simulink model "r2_deng_tvg_rev1_13"  (R2012b)
(part 3 of 65)

      |     mask_enables{ismember(mask_names, 'sample_period')} = 'on';
      | end
      | set_param(gcb, 'MaskEnables', mask_enables);
  speadtime1_offset : Subsystem  Tag=xps:sw_reg  AncestorBlock=xps_library/software register  mask(swreg){io_dir=From Processor, io_delay=1, sample_period=1, names=speadtime_offset1, bitwidths=32, bin_pts=0, arith_types=0, sim_port=on, show_format=on}
      mask prompts: io_dir "I/O direction"; io_delay "I/O delay"; sample_period "Sample period"; names "Bitfield names [msb...lsb]"; bitwidths "Bitfield widths"; bin_pts "Bitfield binary pts"; arith_types "Bitfield types, ufix=0, fix=1, bool=2"; sim_port "Provide sim input/output?"; show_format "Print format string?"
      mask help: A 32-bit software-accessible register. Can be divided into bitfields of varying widths and types using the fields in the block mask.
      mask init:
      | try
      |     swreg_init(gcb)
      | catch ex
      |     disp(sprintf('%s: %s', gcb, ex.message))
      |     errordlg(ex.message)
      | end
      settings: AttributesFormatString=1input:uf32.0 = 32 bits
      mask TypeOptions io_dir: To Processor | From Processor
      mask Callback io_dir:
      | mask_enables = get_param(gcb, 'MaskEnables');
      | mask_names = get_param(gcb, 'MaskNames');
      | if strcmp(get_param(gcb, 'io_dir'), 'To Processor'),
      |     mask_enables{ismember(mask_names, 'sample_period')} = 'off';
      | else
      |     mask_enables{ismember(mask_names, 'sample_period')} = 'on';
      | end
      | set_param(gcb, 'MaskEnables', mask_enables);
  src_sel_cntrl : Subsystem  Tag=xps:sw_reg  AncestorBlock=xps_library/software register  mask(swreg){io_dir=From Processor, io_delay=1, sample_period=1, names=[src_sel_0 src_sel_1], bitwidths=[2 2], bin_pts=[0 0], arith_types=[0 0], sim_port=on, show_format=on}
      mask prompts: io_dir "I/O direction"; io_delay "I/O delay"; sample_period "Sample period"; names "Bitfield names [msb...lsb]"; bitwidths "Bitfield widths"; bin_pts "Bitfield binary pts"; arith_types "Bitfield types, ufix=0, fix=1, bool=2"; sim_port "Provide sim input/output?"; show_format "Print format string?"
      mask help: A 32-bit software-accessible register. Can be divided into bitfields of varying widths and types using the fields in the block mask.
      mask init:
      | try
      |     swreg_init(gcb)
      | catch ex
      |     disp(sprintf('%s: %s', gcb, ex.message))
      |     errordlg(ex.message)
      | end
      settings: AttributesFormatString=2 inputs:uf2.0,uf2.0 = 4 bits
      mask TypeOptions io_dir: To Processor | From Processor
      mask Callback io_dir:
      | mask_enables = get_param(gcb, 'MaskEnables');
      | mask_names = get_param(gcb, 'MaskNames');
      | if strcmp(get_param(gcb, 'io_dir'), 'To Processor'),
      |     mask_enables{ismember(mask_names, 'sample_period')} = 'off';
      | else
      |     mask_enables{ismember(mask_names, 'sample_period')} = 'on';
      | end
      | set_param(gcb, 'MaskEnables', mask_enables);
  ss_fifo_in : Subsystem  Tag=casper:bitsnap  AncestorBlock=casper_library_scopes/bitfield snapshot  mask(bitsnap){io_names=[d0 d1 d2 d3 d4 d5 d6 d7 gpio_trig], io_widths=[10 10 10 10 10 10 10 10 1], io_bps=[9 9 9 9 9 9 9 9 0], io_types=[1 1 1 1 1 1 1 1 2], show_format=on, snap_storage=bram, snap_dram_dimm=2, snap_dram_clock=250, snap_nsamples=9, snap_data_width=128, snap_offset=on, snap_circap=off, snap_value=off, snap_use_dsp48=off, snap_delay=1, extra_names=[c d], extra_widths=[30 2], extra_bps=[0 0], extra_types=[0 0]}
      mask prompts: io_names "Names [msb...lsb]"; io_widths "Bitwidths [msb...lsb]"; io_bps "Binary pts [msb...lsb]"; io_types "Data types [msb...lsb], ufix=0, fix=1, bool=2"; show_format "Print format string?"; snap_storage "Storage medium"; snap_dram_dimm "DRAM dimm"; snap_dram_clock "DRAM clock rate"; snap_nsamples "Number of Samples (2^?)"; snap_data_width "Data width"; snap_offset "Start delay support"; snap_circap "Circular capture support"; snap_value "Extra value capture support"; snap_use_dsp48 "Use DSP48s to implement counters"; snap_delay "Pre-snapshot delay"; extra_names "Names [msb...lsb]"; extra_widths "Widths [msb...lsb]"; extra_bps "Binary pts [msb...lsb]"; extra_types "Data types [msb...lsb], ufix=0, fix=1, bool=2"
      mask help:
      | A wrapped snapshot block. Allows specification of inputs to a snapblock word so the toolflow can automatically set up the scope.
      | See documentation for snapshot for explanation of parameters.
      mask init:
      | bitsnap_init(gcb);
      settings: AttributesFormatString=snap(9):f10.9,f10.9,f10.9,f10.9,f10.9,f10.9,f10.9,f10.9,b = 81 bits
      mask TypeOptions snap_storage: bram | dram
      mask Callback snap_storage: bitsnap_callback();
      mask TypeOptions snap_dram_dimm: 1 | 2 | 3 | 4
      mask TypeOptions snap_dram_clock: 200 | 250 | 266 | 300 | 333
      mask TypeOptions snap_data_width: 8 | 16 | 32 | 64 | 128
      mask Callback snap_value: bitsnap_callback();
  ss_localtime : Subsystem  Tag=casper:bitsnap  AncestorBlock=casper_library_scopes/bitfield snapshot  mask(bitsnap){io_names=time, io_widths=64, io_bps=0, io_types=0, show_format=on, snap_storage=bram, snap_dram_dimm=2, snap_dram_clock=250, snap_nsamples=9, snap_data_width=64, snap_offset=on, snap_circap=off, snap_value=off, snap_use_dsp48=off, snap_delay=1, extra_names=[c d], extra_widths=[30 2], extra_bps=[0 0], extra_types=[0 0]}
      mask prompts: io_names "Names [msb...lsb]"; io_widths "Bitwidths [msb...lsb]"; io_bps "Binary pts [msb...lsb]"; io_types "Data types [msb...lsb], ufix=0, fix=1, bool=2"; show_format "Print format string?"; snap_storage "Storage medium"; snap_dram_dimm "DRAM dimm"; snap_dram_clock "DRAM clock rate"; snap_nsamples "Number of Samples (2^?)"; snap_data_width "Data width"; snap_offset "Start delay support"; snap_circap "Circular capture support"; snap_value "Extra value capture support"; snap_use_dsp48 "Use DSP48s to implement counters"; snap_delay "Pre-snapshot delay"; extra_names "Names [msb...lsb]"; extra_widths "Widths [msb...lsb]"; extra_bps "Binary pts [msb...lsb]"; extra_types "Data types [msb...lsb], ufix=0, fix=1, bool=2"
      mask help:
      | A wrapped snapshot block. Allows specification of inputs to a snapblock word so the toolflow can automatically set up the scope.
      | See documentation for snapshot for explanation of parameters.
      mask init:
      | bitsnap_init(gcb);
      settings: AttributesFormatString=snap(1):uf64.0 = 64 bits
      mask TypeOptions snap_storage: bram | dram
      mask Callback snap_storage: bitsnap_callback();
      mask TypeOptions snap_dram_dimm: 1 | 2 | 3 | 4
      mask TypeOptions snap_dram_clock: 200 | 250 | 266 | 300 | 333
      mask TypeOptions snap_data_width: 8 | 16 | 32 | 64 | 128
      mask Callback snap_value: bitsnap_callback();
  ss_trig_time_lsw : Subsystem  Tag=xps:sw_reg  AncestorBlock=xps_library/software register  mask(swreg){io_dir=From Processor, io_delay=1, sample_period=1, names=reg, bitwidths=32, bin_pts=0, arith_types=0, sim_port=on, show_format=on}
      mask prompts: io_dir "I/O direction"; io_delay "I/O delay"; sample_period "Sample period"; names "Bitfield names [msb...lsb]"; bitwidths "Bitfield widths"; bin_pts "Bitfield binary pts"; arith_types "Bitfield types, ufix=0, fix=1, bool=2"; sim_port "Provide sim input/output?"; show_format "Print format string?"
      mask help: A 32-bit software-accessible register. Can be divided into bitfields of varying widths and types using the fields in the block mask.
      mask init:
      | try
      |     swreg_init(gcb)
      | catch ex
      |     disp(sprintf('%s: %s', gcb, ex.message))
      |     errordlg(ex.message)
      | end
      settings: AttributesFormatString=1input:uf32.0 = 32 bits
      mask TypeOptions io_dir: To Processor | From Processor
      mask Callback io_dir:
      | mask_enables = get_param(gcb, 'MaskEnables');
      | mask_names = get_param(gcb, 'MaskNames');
      | if strcmp(get_param(gcb, 'io_dir'), 'To Processor'),
      |     mask_enables{ismember(mask_names, 'sample_period')} = 'off';
      | else
      |     mask_enables{ismember(mask_names, 'sample_period')} = 'on';
      | end
      | set_param(gcb, 'MaskEnables', mask_enables);
  ss_trig_time_msw : Subsystem  Tag=xps:sw_reg  AncestorBlock=xps_library/software register  mask(swreg){io_dir=From Processor, io_delay=1, sample_period=1, names=reg, bitwidths=32, bin_pts=0, arith_types=0, sim_port=on, show_format=on}
      mask prompts: io_dir "I/O direction"; io_delay "I/O delay"; sample_period "Sample period"; names "Bitfield names [msb...lsb]"; bitwidths "Bitfield widths"; bin_pts "Bitfield binary pts"; arith_types "Bitfield types, ufix=0, fix=1, bool=2"; sim_port "Provide sim input/output?"; show_format "Print format string?"
      mask help: A 32-bit software-accessible register. Can be divided into bitfields of varying widths and types using the fields in the block mask.
      mask init:
      | try
      |     swreg_init(gcb)
      | catch ex
      |     disp(sprintf('%s: %s', gcb, ex.message))
      |     errordlg(ex.message)
      | end
      settings: AttributesFormatString=1input:uf32.0 = 32 bits
      mask TypeOptions io_dir: To Processor | From Processor
      mask Callback io_dir:
      | mask_enables = get_param(gcb, 'MaskEnables');
      | mask_names = get_param(gcb, 'MaskNames');
      | if strcmp(get_param(gcb, 'io_dir'), 'To Processor'),
      |     mask_enables{ismember(mask_names, 'sample_period')} = 'off';
      | else
      |     mask_enables{ismember(mask_names, 'sample_period')} = 'on';
      | end
      | set_param(gcb, 'MaskEnables', mask_enables);
  start_flag_lsw : Subsystem  Tag=xps:sw_reg  AncestorBlock=xps_library/software register  mask(swreg){io_dir=From Processor, io_delay=1, sample_period=1, names=reg, bitwidths=32, bin_pts=0, arith_types=0, sim_port=on, show_format=on}
      mask prompts: io_dir "I/O direction"; io_delay "I/O delay"; sample_period "Sample period"; names "Bitfield names [msb...lsb]"; bitwidths "Bitfield widths"; bin_pts "Bitfield binary pts"; arith_types "Bitfield types, ufix=0, fix=1, bool=2"; sim_port "Provide sim input/output?"; show_format "Print format string?"
      mask help: A 32-bit software-accessible register. Can be divided into bitfields of varying widths and types using the fields in the block mask.
      mask init:
      | try
      |     swreg_init(gcb)
      | catch ex
      |     disp(sprintf('%s: %s', gcb, ex.message))
      |     errordlg(ex.message)
      | end
      settings: AttributesFormatString=1input:uf32.0 = 32 bits
      mask TypeOptions io_dir: To Processor | From Processor
      mask Callback io_dir:
      | mask_enables = get_param(gcb, 'MaskEnables');
      | mask_names = get_param(gcb, 'MaskNames');
      | if strcmp(get_param(gcb, 'io_dir'), 'To Processor'),
      |     mask_enables{ismember(mask_names, 'sample_period')} = 'off';
      | else
      |     mask_enables{ismember(mask_names, 'sample_period')} = 'on';
      | end
      | set_param(gcb, 'MaskEnables', mask_enables);
  start_flag_msw : Subsystem  Tag=xps:sw_reg  AncestorBlock=xps_library/software register  mask(swreg){io_dir=From Processor, io_delay=1, sample_period=1, names=reg, bitwidths=32, bin_pts=0, arith_types=0, sim_port=on, show_format=on}
      mask prompts: io_dir "I/O direction"; io_delay "I/O delay"; sample_period "Sample period"; names "Bitfield names [msb...lsb]"; bitwidths "Bitfield widths"; bin_pts "Bitfield binary pts"; arith_types "Bitfield types, ufix=0, fix=1, bool=2"; sim_port "Provide sim input/output?"; show_format "Print format string?"
      mask help: A 32-bit software-accessible register. Can be divided into bitfields of varying widths and types using the fields in the block mask.
      mask init:
      | try
      |     swreg_init(gcb)
      | catch ex
      |     disp(sprintf('%s: %s', gcb, ex.message))
      |     errordlg(ex.message)
      | end
      settings: AttributesFormatString=1input:uf32.0 = 32 bits
      mask TypeOptions io_dir: To Processor | From Processor
      mask Callback io_dir:
      | mask_enables = get_param(gcb, 'MaskEnables');
      | mask_names = get_param(gcb, 'MaskNames');
      | if strcmp(get_param(gcb, 'io_dir'), 'To Processor'),
      |     mask_enables{ismember(mask_names, 'sample_period')} = 'off';
      | else
      |     mask_enables{ismember(mask_names, 'sample_period')} = 'on';
      | end
      | set_param(gcb, 'MaskEnables', mask_enables);
  start_load_time_lsw : Subsystem  Tag=xps:sw_reg  AncestorBlock=xps_library/software register  mask(swreg){io_dir=From Processor, io_delay=1, sample_period=1, names=reg, bitwidths=32, bin_pts=0, arith_types=0, sim_port=on, show_format=on}
      mask prompts: io_dir "I/O direction"; io_delay "I/O delay"; sample_period "Sample period"; names "Bitfield names [msb...lsb]"; bitwidths "Bitfield widths"; bin_pts "Bitfield binary pts"; arith_types "Bitfield types, ufix=0, fix=1, bool=2"; sim_port "Provide sim input/output?"; show_format "Print format string?"
      mask help: A 32-bit software-accessible register. Can be divided into bitfields of varying widths and types using the fields in the block mask.
      mask init:
      | try
      |     swreg_init(gcb)
      | catch ex
      |     disp(sprintf('%s: %s', gcb, ex.message))
      |     errordlg(ex.message)
      | end
      settings: AttributesFormatString=1input:uf32.0 = 32 bits
      mask TypeOptions io_dir: To Processor | From Processor
      mask Callback io_dir:
      | mask_enables = get_param(gcb, 'MaskEnables');
      | mask_names = get_param(gcb, 'MaskNames');
      | if strcmp(get_param(gcb, 'io_dir'), 'To Processor'),
      |     mask_enables{ismember(mask_names, 'sample_period')} = 'off';
      | else
      |     mask_enables{ismember(mask_names, 'sample_period')} = 'on';
      | end
      | set_param(gcb, 'MaskEnables', mask_enables);
  start_load_time_msw : Subsystem  Tag=xps:sw_reg  AncestorBlock=xps_library/software register  mask(swreg){io_dir=From Processor, io_delay=1, sample_period=1, names=reg, bitwidths=32, bin_pts=0, arith_types=0, sim_port=on, show_format=on}
      mask prompts: io_dir "I/O direction"; io_delay "I/O delay"; sample_period "Sample period"; names "Bitfield names [msb...lsb]"; bitwidths "Bitfield widths"; bin_pts "Bitfield binary pts"; arith_types "Bitfield types, ufix=0, fix=1, bool=2"; sim_port "Provide sim input/output?"; show_format "Print format string?"
      mask help: A 32-bit software-accessible register. Can be divided into bitfields of varying widths and types using the fields in the block mask.
      mask init:
      | try
      |     swreg_init(gcb)
      | catch ex
      |     disp(sprintf('%s: %s', gcb, ex.message))
      |     errordlg(ex.message)
      | end
      settings: AttributesFormatString=1input:uf32.0 = 32 bits
      mask TypeOptions io_dir: To Processor | From Processor
      mask Callback io_dir:
      | mask_enables = get_param(gcb, 'MaskEnables');
      | mask_names = get_param(gcb, 'MaskNames');
      | if strcmp(get_param(gcb, 'io_dir'), 'To Processor'),
      |     mask_enables{ismember(mask_names, 'sample_period')} = 'off';
      | else
      |     mask_enables{ismember(mask_names, 'sample_period')} = 'on';
      | end
      | set_param(gcb, 'MaskEnables', mask_enables);
  start_time_lsw : Subsystem  Tag=xps:sw_reg  AncestorBlock=xps_library/software register  mask(swreg){io_dir=From Processor, io_delay=1, sample_period=1, names=reg, bitwidths=32, bin_pts=0, arith_types=0, sim_port=on, show_format=on}
      mask prompts: io_dir "I/O direction"; io_delay "I/O delay"; sample_period "Sample period"; names "Bitfield names [msb...lsb]"; bitwidths "Bitfield widths"; bin_pts "Bitfield binary pts"; arith_types "Bitfield types, ufix=0, fix=1, bool=2"; sim_port "Provide sim input/output?"; show_format "Print format string?"
      mask help: A 32-bit software-accessible register. Can be divided into bitfields of varying widths and types using the fields in the block mask.
      mask init:
      | try
      |     swreg_init(gcb)
      | catch ex
      |     disp(sprintf('%s: %s', gcb, ex.message))
      |     errordlg(ex.message)
      | end
      settings: AttributesFormatString=1input:uf32.0 = 32 bits
      mask TypeOptions io_dir: To Processor | From Processor
      mask Callback io_dir:
      | mask_enables = get_param(gcb, 'MaskEnables');
      | mask_names = get_param(gcb, 'MaskNames');
      | if strcmp(get_param(gcb, 'io_dir'), 'To Processor'),
      |     mask_enables{ismember(mask_names, 'sample_period')} = 'off';
      | else
      |     mask_enables{ismember(mask_names, 'sample_period')} = 'on';
      | end
      | set_param(gcb, 'MaskEnables', mask_enables);
  start_time_msw : Subsystem  Tag=xps:sw_reg  AncestorBlock=xps_library/software register  mask(swreg){io_dir=From Processor, io_delay=1, sample_period=1, names=reg, bitwidths=32, bin_pts=0, arith_types=0, sim_port=on, show_format=on}
      mask prompts: io_dir "I/O direction"; io_delay "I/O delay"; sample_period "Sample period"; names "Bitfield names [msb...lsb]"; bitwidths "Bitfield widths"; bin_pts "Bitfield binary pts"; arith_types "Bitfield types, ufix=0, fix=1, bool=2"; sim_port "Provide sim input/output?"; show_format "Print format string?"
      mask help: A 32-bit software-accessible register. Can be divided into bitfields of varying widths and types using the fields in the block mask.
      mask init:
      | try
      |     swreg_init(gcb)
      | catch ex
      |     disp(sprintf('%s: %s', gcb, ex.message))
      |     errordlg(ex.message)
      | end
      settings: AttributesFormatString=1input:uf32.0 = 32 bits
      mask TypeOptions io_dir: To Processor | From Processor
      mask Callback io_dir:
      | mask_enables = get_param(gcb, 'MaskEnables');
      | mask_names = get_param(gcb, 'MaskNames');
      | if strcmp(get_param(gcb, 'io_dir'), 'To Processor'),
      |     mask_enables{ismember(mask_names, 'sample_period')} = 'off';
      | else
      |     mask_enables{ismember(mask_names, 'sample_period')} = 'on';
      | end
      | set_param(gcb, 'MaskEnables', mask_enables);
  stop_load_time_lsw : Subsystem  Tag=xps:sw_reg  AncestorBlock=xps_library/software register  mask(swreg){io_dir=From Processor, io_delay=1, sample_period=1, names=reg, bitwidths=32, bin_pts=0, arith_types=0, sim_port=on, show_format=on}
      mask prompts: io_dir "I/O direction"; io_delay "I/O delay"; sample_period "Sample period"; names "Bitfield names [msb...lsb]"; bitwidths "Bitfield widths"; bin_pts "Bitfield binary pts"; arith_types "Bitfield types, ufix=0, fix=1, bool=2"; sim_port "Provide sim input/output?"; show_format "Print format string?"
      mask help: A 32-bit software-accessible register. Can be divided into bitfields of varying widths and types using the fields in the block mask.
      mask init:
      | try
      |     swreg_init(gcb)
      | catch ex
      |     disp(sprintf('%s: %s', gcb, ex.message))
      |     errordlg(ex.message)
      | end
      settings: AttributesFormatString=1input:uf32.0 = 32 bits
      mask TypeOptions io_dir: To Processor | From Processor
      mask Callback io_dir:
      | mask_enables = get_param(gcb, 'MaskEnables');
      | mask_names = get_param(gcb, 'MaskNames');
      | if strcmp(get_param(gcb, 'io_dir'), 'To Processor'),
      |     mask_enables{ismember(mask_names, 'sample_period')} = 'off';
      | else
      |     mask_enables{ismember(mask_names, 'sample_period')} = 'on';
      | end
      | set_param(gcb, 'MaskEnables', mask_enables);
  stop_load_time_msw : Subsystem  Tag=xps:sw_reg  AncestorBlock=xps_library/software register  mask(swreg){io_dir=From Processor, io_delay=1, sample_period=1, names=reg, bitwidths=32, bin_pts=0, arith_types=0, sim_port=on, show_format=on}
      mask prompts: io_dir "I/O direction"; io_delay "I/O delay"; sample_period "Sample period"; names "Bitfield names [msb...lsb]"; bitwidths "Bitfield widths"; bin_pts "Bitfield binary pts"; arith_types "Bitfield types, ufix=0, fix=1, bool=2"; sim_port "Provide sim input/output?"; show_format "Print format string?"
      mask help: A 32-bit software-accessible register. Can be divided into bitfields of varying widths and types using the fields in the block mask.
      mask init:
      | try
      |     swreg_init(gcb)
      | catch ex
      |     disp(sprintf('%s: %s', gcb, ex.message))
      |     errordlg(ex.message)
      | end
      settings: AttributesFormatString=1input:uf32.0 = 32 bits
      mask TypeOptions io_dir: To Processor | From Processor
      mask Callback io_dir:
      | mask_enables = get_param(gcb, 'MaskEnables');
      | mask_names = get_param(gcb, 'MaskNames');
      | if strcmp(get_param(gcb, 'io_dir'), 'To Processor'),
      |     mask_enables{ismember(mask_names, 'sample_period')} = 'off';
      | else
      |     mask_enables{ismember(mask_names, 'sample_period')} = 'on';
      | end
      | set_param(gcb, 'MaskEnables', mask_enables);
  tick_offset_lsw : Subsystem  Tag=xps:sw_reg  AncestorBlock=xps_library/software register  mask(swreg){io_dir=From Processor, io_delay=1, sample_period=1, names=reg, bitwidths=32, bin_pts=0, arith_types=0, sim_port=off, show_format=on}
      mask prompts: io_dir "I/O direction"; io_delay "I/O delay"; sample_period "Sample period"; names "Bitfield names [msb...lsb]"; bitwidths "Bitfield widths"; bin_pts "Bitfield binary pts"; arith_types "Bitfield types, ufix=0, fix=1, bool=2"; sim_port "Provide sim input/output?"; show_format "Print format string?"
      mask help: A 32-bit software-accessible register. Can be divided into bitfields of varying widths and types using the fields in the block mask.
      mask init:
      | try
      |     swreg_init(gcb)
      | catch ex
      |     disp(sprintf('%s: %s', gcb, ex.message))
      |     errordlg(ex.message)
      | end
      settings: AttributesFormatString=1input:uf32.0 = 32 bits
      mask TypeOptions io_dir: To Processor | From Processor
      mask Callback io_dir:
      | mask_enables = get_param(gcb, 'MaskEnables');
      | mask_names = get_param(gcb, 'MaskNames');
      | if strcmp(get_param(gcb, 'io_dir'), 'To Processor'),
      |     mask_enables{ismember(mask_names, 'sample_period')} = 'off';
      | else
      |     mask_enables{ismember(mask_names, 'sample_period')} = 'on';
      | end
      | set_param(gcb, 'MaskEnables', mask_enables);
  tick_offset_msw : Subsystem  Tag=xps:sw_reg  AncestorBlock=xps_library/software register  mask(swreg){io_dir=From Processor, io_delay=1, sample_period=1, names=reg, bitwidths=32, bin_pts=0, arith_types=0, sim_port=off, show_format=on}
      mask prompts: io_dir "I/O direction"; io_delay "I/O delay"; sample_period "Sample period"; names "Bitfield names [msb...lsb]"; bitwidths "Bitfield widths"; bin_pts "Bitfield binary pts"; arith_types "Bitfield types, ufix=0, fix=1, bool=2"; sim_port "Provide sim input/output?"; show_format "Print format string?"
      mask help: A 32-bit software-accessible register. Can be divided into bitfields of varying widths and types using the fields in the block mask.
      mask init:
      | try
      |     swreg_init(gcb)
      | catch ex
      |     disp(sprintf('%s: %s', gcb, ex.message))
      |     errordlg(ex.message)
      | end
      settings: AttributesFormatString=1input:uf32.0 = 32 bits
      mask TypeOptions io_dir: To Processor | From Processor
      mask Callback io_dir:
      | mask_enables = get_param(gcb, 'MaskEnables');
      | mask_names = get_param(gcb, 'MaskNames');
      | if strcmp(get_param(gcb, 'io_dir'), 'To Processor'),
      |     mask_enables{ismember(mask_names, 'sample_period')} = 'off';
      | else
      |     mask_enables{ismember(mask_names, 'sample_period')} = 'on';
      | end
      | set_param(gcb, 'MaskEnables', mask_enables);
  ticks_since_mrst : Subsystem
  tvg_spead_time_with_pkt_ctr : Subsystem  mask{packetlen_bits=9}
      mask prompts: packetlen_bits "Packet length, num 80-bit words (2^?):"
  wng0 : Subsystem
  wng1 : Subsystem
  wng_corr : Subsystem
  wng_rst : Subsystem
  xsg : xps_library/XSG core config  Tag=xps:xsg  hw_sys=ROACH2:sx475t  clk_src=sys_clk  ROACH_clk_src=sys_clk  ROACH2_clk_src=sys_clk  MKDIG_clk_src=sys_clk  clk_rate=1712/8  sample_period=1  synthesis_tool=XST
  tag scope: arb_en0=global, arb_rst0=global, dram_addr_offset0=global, dram_rd_repeat0=global, dram_rd_repeat_delay0=global, dram_rd_trig0=global, dram_read_length0=global, dram_tvg0=global, dram_tvg_length0=global, local_time=global, spead_data0=global, spead_data1=global, spead_data2=global, spead_data3=global, spead_eof0=global, spead_eof1=global, spead_eof2=global, spead_eof3=global, spead_valid0=global, spead_valid1=global, spead_valid2=global, spead_valid3=global, tvg_sel0=global
  wires:
  [tvg_select0] -> Delay102/1
  Mux/1 -> Assert/1  "d80_0"
  fifo0/1(fifo_data80) -> pipeline96/1(d)  "data00"
  fifo0/2(fifo_dv) -> pipeline97/1(d)  "dv00"
  fifo0/3(word_start) -> pipeline98/1(d)  "ws00"
  fifo0/4(pkt_start) -> pipeline99/1(d)  "ps00"
  gbe_porttx/1(in_reg) -> pipeline16/1(d), pipeline15/1(d)
  Constant9/1 -> gbe_porttx/1(sim_1)
  Constant10/1 -> gbe_iptx0/1(sim_1)
  Constant12/1 -> gbe_iptx1/1(sim_1)
  Constant13/1 -> gbe_iptx2/1(sim_1)
  Constant14/1 -> gbe_iptx3/1(sim_1)
  Constant15/1 -> digitiser_id/1(sim_1)
  Constant17/1 -> receptor_id/1(sim_1)
  fifo0/5(fifo_full) -> Terminator16/1  "full00"
  fifo0/6(fifo_empty) -> Terminator23/1  "empty00"
  fifo1/1(fifo_data80) -> pipeline100/1(d)  "data01"
  fifo1/2(fifo_dv) -> pipeline101/1(d)  "dv01"
  fifo1/3(word_start) -> pipeline102/1(d)  "ws01"
  fifo1/4(pkt_start) -> pipeline103/1(d)  "ps01"
  pack_80_64_1/3(data64) -> pipeline117/1(d)  "d64_00"
  pack_80_64_1/2(valid64) -> pipeline116/1(d)  "v64_01"
  pack_80_64_1/1(ready64) -> pipeline115/1(d)  "r64_01"
  fifo1/5(fifo_full) -> Terminator18/1
  fifo1/6(fifo_empty) -> Terminator20/1
  Constant16/1 -> digitiser_id/2(sim_2)
  receptor_id/1(in_receptor_id) -> bus_create/3(in3)
  Constant6/1 -> receptor_id/2(sim_2)
  Constant19/1 -> receptor_id/3(sim_3)
  [hdr_0x3101] -> bus_create9/1(in1)
  [pol0_id] -> bus_create9/2(in2)
  [hdr_0x3101] -> bus_create1/1(in1)
  [pol0_id] -> bus_create1/2(in2)
  [speadtime0] -> spead_pack0/8(hdr5_0x1600_DIR), spead_pack0/4(hdr_heap_id)  "timein0"
  bus_create9/1(bus_out) -> spead_pack0/9(hdr6_0x3101_DIR)
  [status0] -> spead_pack0/10(hdr7_0x3102_DIR)
  bus_create1/1(bus_out) -> spead_pack1/9(hdr6_0x3101_DIR)
  [status1] -> spead_pack1/10(hdr7_0x3102_DIR)
  [tvg_ltime] -> fifo_select/1(localtime)
  fifo_select/1(select) -> Delay3/1  "fifo_select"
  Delay3/1 -> Logical18/2, Logical18/1, Gateway Out4/1  "fifoselect"
  [speadtime1] -> spead_pack1/4(hdr_heap_id), spead_pack1/8(hdr5_0x1600_DIR)  "timein1"
  pack_80_64_00/1(ready64) -> pipeline112/1(d)  "r64_00"
  pack_80_64_00/2(valid64) -> pipeline113/1(d)  "v64_00"
  pack_80_64_00/3(data64) -> pipeline114/1(d)  "d64_00"
  [spead_heapsize] -> spead_pack0/5(hdr_heap_size)
  [spead_heapoffset] -> spead_pack0/6(hdr_heap_offset)
  [spead_pktlen] -> spead_pack0/7(hdr_pkt_len_words)
  [spead_heapsize] -> spead_pack1/5(hdr_heap_size)
  [spead_heapoffset] -> spead_pack1/6(hdr_heap_offset)
  [spead_pktlen] -> spead_pack1/7(hdr_pkt_len_words)
  [masked_time] -> Delay128/1
  Assert/1 -> [fifo0_data], fifo1/1(data80), fifo0/1(data80)
  tvg_spead_time_with_pkt_ctr/1(local_time) -> Delay131/1
  tvg_spead_time_with_pkt_ctr/3(tvg_data_pol0) -> Delay133/1
  tvg_spead_time_with_pkt_ctr/4(tvg_data_pol1) -> Delay134/1
  tvg_spead_time_with_pkt_ctr/2(spead_time) -> Delay132/1
  spead_pack1/4(data_overflow) -> Terminator15/1
  [adc_data_offset] -> spead_pack0/11(hdr8_0x3300)
  [adc_data_offset] -> spead_pack1/11(hdr8_0x3300)
  Constant26/1 -> [spead_heapsize]
  Constant27/1 -> [spead_pktlen]
  Constant45/1 -> [spead_heapoffset]
  spead_pack0/4(data_overflow) -> Terminator12/1
  spead_pack0/3(eof) -> pipeline56/1(d)
  spead_pack0/1(data_out) -> pipeline54/1(d)  "packd"
  spead_pack0/2(valid_out) -> pipeline55/1(d)  "packv"
  spead_pack1/1(data_out) -> pipeline57/1(d)
  spead_pack1/2(valid_out) -> pipeline58/1(d)
  spead_pack1/3(eof) -> pipeline59/1(d)
  [fifoselect] -> edge_detect5/1(in), Inverter2/1
  Register5/1 -> [speadtime0]  "speadtime0"
  Inverter2/1 -> edge_detect6/1(in)
  edge_detect5/1(out) -> Register5/2
  edge_detect6/1(out) -> Register6/2
  Register6/1 -> [speadtime1]  "speadtime1"
  Constant8/1 -> [adc_data_offset]
  [mrst] -> ticks_since_mrst/1(reset)
  [sync] -> ticks_since_mrst/2(sync)
  ticks_since_mrst/1(time64) -> slice3/1, [local_time]  "localtime"
  [msync] -> [sync]  "sync"
  edge_detect2/1(out) -> [mrst]  "mrst"
  edge_detect1/1(out) -> [msync]  "msync"
  edge_detect4/1(out) -> [clr_status]  "clr_status"
  [local_time] -> slice1/1, slice2/1
  Constant28/1 -> control/3(sim_3)
  Constant44/1 -> control/1(sim_1)
  Constant24/1 -> control/2(sim_2)
  Constant33/1 -> control/6(sim_6)
  Constant30/1 -> control/5(sim_5)
  Constant36/1 -> control/4(sim_4)
  Pulse Generator/1 -> control/8(sim_8)
  [tick_offset] -> ticks_since_mrst/3(offset)
  edge_detect10/1(out) -> [load_tick_offset]  "mrst"
  Constant20/1 -> control/9(sim_9)
  digitiser_id/1(in_digitiser_serial) -> bus_create/1(in1)
  digitiser_id/2(in_digitiser_type) -> bus_create/2(in2)
  Constant43/1 -> flag_setup/3(sim_3)
  Constant42/1 -> flag_setup/2(sim_2)
  Constant39/1 -> flag_setup/1(sim_1)
  Counter Free-Running3/1 -> Relational Operator4/2
  Constant48/1 -> Relational Operator4/1
  Relational Operator4/1 -> flag_setup/4(sim_4)
  Constant52/1 -> start_flag_msw/1(sim_1)
  Constant53/1 -> start_flag_lsw/1(sim_1)
  Constant51/1 -> end_flag_msw/1(sim_1)
  Constant50/1 -> end_flag_lsw/1(sim_1)
  Concat4/1 -> Delay49/1  "starttime"
  Concat5/1 -> Delay50/1  "stoptime"
  [flag_start_time] -> Delay46/1
  [local_time] -> Delay45/1, Delay47/1
  [flag_end_time] -> Delay48/1, Delay51/1
  Relational/1 -> Logical2/2  "start_okay"
  [flag_armed] -> Delay44/1
  Relational1/1 -> Logical4/2  "end_okay"
  Logical2/1 -> Delay23/1  "start_okay"
  Logical4/1 -> Logical3/1  "end_okay"
  edge_detect9/1(out) -> [load_flag_time]  "loadtimes"
  Constant4/1 -> Register1/1
  edge_detect8/1(out) -> [reset_flag_time]  "rst"
  [reset_flag_time] -> Register1/2
  [load_flag_time] -> Register1/3
  Register1/1 -> [flag_armed]  "armed"
  Relational Operator3/1 -> flag_setup/5(sim_5)
  Relational2/1 -> Delay22/1  "zero_stop"
  Constant2/1 -> Relational2/2
  Logical3/1 -> Logical1/2  "eokay"
  Counter Free-Running2/1 -> Relational Operator3/2
  Constant5/1 -> Relational Operator3/1
  Logical5/1 -> sample_masking/2(den_in)
  Constant49/1 -> start_time_msw/1(sim_1)
  Constant54/1 -> start_time_lsw/1(sim_1)
  Constant3/1 -> end_time_msw/1(sim_1)
  Constant11/1 -> end_time_lsw/1(sim_1)
  Relational3/1 -> Logical6/2  "start_okay"
  Relational4/1 -> Logical8/2  "end_okay"
  [start_time] -> Delay39/1
  Relational6/1 -> Delay15/1  "first_sample"
  [end_time] -> Delay41/1
  Relational7/1 -> Delay16/1  "last_sample"
  [sample_end] -> sample_masking/6(sample_end)
  [sample_start] -> sample_masking/5(sample_start)
  sample_masking/2(den_out) -> Delay126/1  "enable"
  sample_masking/3(data_mask) -> Delay127/1  "mask"
  edge_detect11/1(out) -> [reset_en_time]  "reset_en_time"
  Relational Operator5/1 -> control_output/2(sim_2)
  Counter Free-Running4/1 -> Relational Operator6/2, Relational Operator5/2
  Constant38/1 -> Relational Operator5/1
  edge_detect12/1(out) -> [load_en_time]  "load_en_time"
  Concat/1 -> Delay42/1
  Concat1/1 -> Delay43/1
  Constant22/1 -> Register2/1
  [reset_en_time] -> Register2/2
  [load_en_time] -> Register2/3
  Register2/1 -> [en_armed]  "armed"
  Logical6/1 -> Delay17/1  "start_okay"
  Logical8/1 -> Logical7/1  "end_okay"
  Logical7/1 -> Logical5/2
  Constant34/1 -> Delay37/1
  Relational5/1 -> Delay14/1
  Constant29/1 -> control_output/3(sim_3)
  Constant47/1 -> control_output/4(sim_4)
  Constant31/1 -> Relational Operator6/1
  Relational Operator6/1 -> control_output/1(sim_1)
  [data_enable] -> Delay129/1
  [sample_mask] -> Delay130/1
  Concat2/1 -> Register3/1
  [load_tick_offset] -> Register3/2
  Register3/1 -> [tick_offset]
  fifo2/1(fifo_data80) -> pipeline104/1(d)  "data00"
  fifo2/2(fifo_dv) -> pipeline105/1(d)  "dv00"
  fifo2/3(word_start) -> pipeline106/1(d)  "ws00"
  fifo2/4(pkt_start) -> pipeline107/1(d)  "ps00"
  fifo2/5(fifo_full) -> Terminator3/1  "full00"
  fifo2/6(fifo_empty) -> Terminator6/1  "empty00"
  fifo3/1(fifo_data80) -> pipeline108/1(d)  "data01"
  fifo3/2(fifo_dv) -> pipeline109/1(d)  "dv01"
  fifo3/3(word_start) -> pipeline110/1(d)  "ws01"
  fifo3/4(pkt_start) -> pipeline111/1(d)  "ps01"
  pack_80_64_3/3(data64) -> pipeline123/1(d)  "d64_00"
  pack_80_64_3/2(valid64) -> pipeline122/1(d)  "v64_01"
  pack_80_64_3/1(ready64) -> pipeline121/1(d)  "r64_01"
  fifo3/5(fifo_full) -> Terminator4/1
  fifo3/6(fifo_empty) -> Terminator5/1
  [hdr_0x3101] -> bus_create3/1(in1)
  [pol1_id] -> bus_create3/2(in2)
  [hdr_0x3101] -> bus_create2/1(in1)
  [pol1_id] -> bus_create2/2(in2)
  [speadtime0] -> spead_pack2/4(hdr_heap_id), spead_pack2/8(hdr5_0x1600_DIR)  "timein0"
  bus_create3/1(bus_out) -> spead_pack2/9(hdr6_0x3101_DIR)
  [status2] -> spead_pack2/10(hdr7_0x3102_DIR)
  bus_create2/1(bus_out) -> spead_pack3/9(hdr6_0x3101_DIR)
  [status3] -> spead_pack3/10(hdr7_0x3102_DIR)
  [speadtime1] -> spead_pack3/8(hdr5_0x1600_DIR), spead_pack3/4(hdr_heap_id)  "timein1"
  pack_80_64_2/1(ready64) -> pipeline118/1(d)  "r64_00"
  pack_80_64_2/2(valid64) -> pipeline119/1(d)  "v64_00"
  pack_80_64_2/3(data64) -> pipeline120/1(d)  "d64_00"
  [spead_heapsize] -> spead_pack2/5(hdr_heap_size)
  [spead_heapoffset] -> spead_pack2/6(hdr_heap_offset)
  [spead_pktlen] -> spead_pack2/7(hdr_pkt_len_words)
  [spead_heapsize] -> spead_pack3/5(hdr_heap_size)
  [spead_heapoffset] -> spead_pack3/6(hdr_heap_offset)
  [spead_pktlen] -> spead_pack3/7(hdr_pkt_len_words)
  spead_pack3/4(data_overflow) -> Terminator2/1
  [adc_data_offset] -> spead_pack2/11(hdr8_0x3300)
  [adc_data_offset] -> spead_pack3/11(hdr8_0x3300)
  spead_pack2/4(data_overflow) -> Terminator1/1
  spead_pack2/3(eof) -> pipeline62/1(d)
  spead_pack2/1(data_out) -> pipeline60/1(d)  "packd"
  spead_pack2/2(valid_out) -> pipeline61/1(d)  "packv"
  spead_pack3/1(data_out) -> pipeline63/1(d)
  spead_pack3/2(valid_out) -> pipeline64/1(d)
  spead_pack3/3(eof) -> pipeline65/1(d)
  Inverter1/1 -> fifo3/2(fifo_we_en)
  [tvg_select1] -> Delay106/1
  Mux1/1 -> Assert1/1  "d80_0"
  [data_80_1] -> Delay109/1
  [tvg_pol1] -> Delay108/1
  Assert1/1 -> fifo3/1(data80), fifo2/1(data80)
  [fifoselect] -> Inverter1/1, fifo2/2(fifo_we_en)
  [gbe_txen_gate0] -> Logical10/2, Logical13/1
  Logical10/1 -> Gateway Out23/1, pipeline86/1(d)
  [gbe_port0] -> gbe0/5(tx_dest_port)
  Constant56/1 -> gbe0/8(rx_overrun_ack), gbe0/7(rx_ack)
  [spead_valid0] -> Logical10/1
  pipeline83/1(q) -> gbe0/2(tx_data)
  [gbe_ip0] -> gbe0/4(tx_dest_ip)
  [gbe_rst] -> pipeline68/1(d)
  [gbe_txen_gate1] -> Logical9/2, Logical14/1
  Logical9/1 -> pipeline85/1(d)
  [gbe_port1] -> gbe1/5(tx_dest_port)
  Constant18/1 -> gbe1/8(rx_overrun_ack), gbe1/7(rx_ack)
  pipeline80/1(q) -> gbe1/2(tx_data)
  [gbe_ip1] -> gbe1/4(tx_dest_ip)
  [gbe_rst] -> pipeline70/1(d)
  [gbe_txen_gate2] -> Logical15/1, Logical12/2
  Logical12/1 -> pipeline82/1(d)
  [gbe_port2] -> gbe2/5(tx_dest_port)
  Constant25/1 -> gbe2/8(rx_overrun_ack), gbe2/7(rx_ack)
  [spead_valid2] -> Logical12/1
  pipeline77/1(q) -> gbe2/2(tx_data)
  [gbe_ip2] -> gbe2/4(tx_dest_ip)
  [gbe_txen_gate3] -> Logical11/2, Logical16/1
  Logical11/1 -> pipeline75/1(d)
  [gbe_port3] -> gbe3/5(tx_dest_port)
  Constant21/1 -> gbe3/8(rx_overrun_ack), gbe3/7(rx_ack)
  [spead_data3] -> pipeline74/1(d)
  [gbe_ip3] -> gbe3/4(tx_dest_ip)
  [clr_status] -> pipeline69/1(d)
  [clr_status] -> pipeline71/1(d)
  [spead_eof0] -> Logical13/2
  [spead_eof1] -> Logical14/2
  Logical15/1 -> pipeline87/1(d)
  [spead_eof2] -> Logical15/2
  Logical16/1 -> pipeline76/1(d)
  [spead_eof3] -> Logical16/2
  gbe0/2(led_rx) -> Terminator77/1
  gbe0/3(led_tx) -> Terminator67/1
  gbe0/4(tx_afull) -> Terminator72/1
  gbe0/5(tx_overflow) -> Terminator73/1
  gbe0/6(rx_data) -> Terminator75/1
  gbe0/7(rx_valid) -> Terminator66/1
  gbe0/8(rx_source_ip) -> Terminator68/1
  gbe0/9(rx_source_port) -> Terminator69/1
  gbe0/10(rx_end_of_frame) -> Terminator70/1
  gbe0/11(rx_bad_frame) -> Terminator71/1
  gbe0/12(rx_overrun) -> Terminator74/1
  gbe0/13(rx_dest_ip) -> Terminator76/1
  gbe1/2(led_rx) -> Terminator13/1
  gbe1/3(led_tx) -> Terminator8/1
  gbe1/4(tx_afull) -> Terminator40/1
  gbe1/5(tx_overflow) -> Terminator43/1
  gbe1/6(rx_data) -> Terminator10/1
  gbe1/7(rx_valid) -> Terminator7/1
  gbe1/8(rx_source_ip) -> Terminator9/1
  gbe1/9(rx_source_port) -> Terminator34/1
  gbe1/10(rx_end_of_frame) -> Terminator37/1
  gbe1/11(rx_bad_frame) -> Terminator38/1
  gbe1/12(rx_overrun) -> Terminator46/1
  gbe1/13(rx_dest_ip) -> Terminator11/1
  gbe2/2(led_rx) -> Terminator21/1
  gbe2/3(led_tx) -> Terminator22/1
  gbe2/5(tx_overflow) -> Terminator29/1
  gbe2/6(rx_data) -> Terminator17/1
  gbe2/7(rx_valid) -> Terminator14/1
  gbe2/8(rx_source_ip) -> Terminator24/1
  gbe2/9(rx_source_port) -> Terminator25/1
  gbe2/10(rx_end_of_frame) -> Terminator26/1
  gbe2/11(rx_bad_frame) -> Terminator27/1
  gbe2/12(rx_overrun) -> Terminator30/1
  gbe2/13(rx_dest_ip) -> Terminator19/1
  gbe3/2(led_rx) -> Terminator35/1
  gbe3/3(led_tx) -> Terminator36/1
  gbe3/4(tx_afull) -> Terminator45/1
  gbe3/5(tx_overflow) -> Terminator47/1
  gbe3/6(rx_data) -> Terminator32/1
  gbe3/7(rx_valid) -> Terminator31/1
  gbe3/8(rx_source_ip) -> Terminator39/1
  gbe3/9(rx_source_port) -> Terminator41/1
  gbe3/10(rx_end_of_frame) -> Terminator42/1
  gbe3/11(rx_bad_frame) -> Terminator44/1
  gbe3/12(rx_overrun) -> Terminator48/1
  gbe3/13(rx_dest_ip) -> Terminator33/1
  Logical13/1 -> pipeline84/1(d)
  Logical14/1 -> pipeline81/1(d)
  [spead_data0] -> pipeline83/1(d)
  [spead_data1] -> pipeline80/1(d)
  [spead_data2] -> pipeline77/1(d)
  [spead_valid3] -> Logical11/1
  scale_wng1/1(in_scale) -> Gateway Out6/1, pipeline43/1(d)
  scale_wng_corr/1(in_scale) -> pipeline42/1(d)
  wng0/1(bus_out) -> [wng0_tp0], pipeline78/1(d)
  wng1/1(bus_out) -> [wng1_tp0], pipeline89/1(d)
  cwg_corr/1(bus_out) -> pipeline91/1(d), pipeline92/1(d), [Bus_expand_cwg_corr]
  bus_addsub/1(dout) -> Delay105/1
  bus_addsub2/1(dout) -> Delay6/1
  bus_addsub3/1(dout) -> Delay9/1
  bus_addsub1/1(dout) -> Delay5/1
  bus_addsub4/1(dout) -> bus_convert6/1(din)
  bus_mult/1(a*b) -> [cwg0_tp1], bus_convert/1(din)
  bus_addsub5/1(dout) -> bus_convert7/1(din)
  bus_mult1/1(a*b) -> bus_convert1/1(din), [cwg1_tp1]
  scale_out1/1(in_scale) -> Gateway Out3/1, pipeline52/1(d)
  Constant35/1 -> scale_wng0/1(sim_1)
  Constant1/1 -> scale_wng_corr/1(sim_1)
  pipeline21/1(q) -> edge_detect12/1(in)
  pipeline22/1(q) -> edge_detect11/1(in)
  pipeline23/1(q) -> [sample_start]
  pipeline24/1(q) -> [sample_end]
  Delay42/1 -> [start_time]
  Delay43/1 -> [end_time]
  Delay49/1 -> [flag_start_time]
  Delay50/1 -> [flag_end_time]
  pipeline41/1(q) -> wng0/1(scale_16_14)
  pipeline42/1(q) -> wng_corr/1(scale_16_14)
  pipeline43/1(q) -> wng1/1(scale_16_14)
  pipeline10/1(q) -> [gbe_ip3]
  pipeline11/1(q) -> [gbe_ip2]
  pipeline13/1(q) -> [gbe_ip0]
  pipeline9/1(q) -> [gbe_port0]
  Delay102/1 -> Mux/1
  Delay103/1 -> Mux/2
  Delay104/1 -> Mux/3
  Delay106/1 -> Mux1/1
  Delay126/1 -> [data_enable]
  Delay127/1 -> [sample_mask]
  Delay128/1 -> tvg_spead_time_with_pkt_ctr/1(localtime64)
  Delay129/1 -> tvg_spead_time_with_pkt_ctr/2(data_enable)
  Delay130/1 -> tvg_spead_time_with_pkt_ctr/3(data_mask)
  Delay131/1 -> [tvg_ltime]
  Delay132/1 -> [tvg_stime]
  Delay133/1 -> [tvg_pol0]
  Delay134/1 -> [tvg_pol1]
  [tvg_pol0] -> Delay103/1
  [data_80_0] -> Delay104/1
  Delay109/1 -> Mux1/3
  Delay108/1 -> Mux1/2
  Delay105/1 -> bus_convert2/1(din)
  Delay5/1 -> bus_convert3/1(din)
  Delay6/1 -> bus_convert4/1(din)
  Delay9/1 -> bus_convert5/1(din)
  Delay139/1 -> bus_addsub4/1(a)
  Delay7/1 -> bus_addsub5/1(a)
  Delay8/1 -> bus_addsub5/2(b)
  pipeline25/1(q) -> Concat/1
  pipeline26/1(q) -> Concat/2
  pipeline27/1(q) -> Concat1/1
  pipeline28/1(q) -> Concat1/2
  pipeline29/1(q) -> [hdr_0x3101]
  pipeline30/1(q) -> [pol0_id]
  pipeline31/1(q) -> [pol1_id]
  control/1(in_up_cnt_rst) -> pipeline/1(d)
  pipeline/1(q) -> edge_detect3/1(in)
  control/2(in_tvg_select0) -> pipeline1/1(d)
  control/3(in_tvg_select1) -> pipeline2/1(d)
  control/4(in_clr_status) -> pipeline3/1(d)
  control/5(in_gbe_rst) -> pipeline4/1(d)
  control/6(in_gbe_txen) -> pipeline5/1(d)
  control/7(in_msync) -> pipeline6/1(d)
  control/8(in_mrst) -> pipeline7/1(d)
  control/9(in_load_tick_offset) -> pipeline8/1(d)
  pipeline8/1(q) -> edge_detect10/1(in)
  pipeline7/1(q) -> edge_detect2/1(in)
  pipeline6/1(q) -> edge_detect1/1(in)
  pipeline4/1(q) -> [gbe_rst]
  pipeline3/1(q) -> edge_detect4/1(in)
  pipeline2/1(q) -> [tvg_select1]
  pipeline1/1(q) -> [tvg_select0]
  pipeline12/1(q) -> [gbe_ip1]
  pipeline16/1(q) -> pipeline124/1(d), pipeline125/1(d)
  pipeline14/1(q) -> [gbe_port1]
  gbe_iptx0/1(in_reg) -> pipeline13/1(d)
  gbe_iptx1/1(in_reg) -> pipeline12/1(d)
  gbe_iptx2/1(in_reg) -> pipeline11/1(d)
  gbe_iptx3/1(in_reg) -> pipeline10/1(d)
  pipeline17/1(q) -> Concat2/1
  tick_offset_lsw/1(in_reg) -> pipeline18/1(d)
  pipeline18/1(q) -> Concat2/2
  slice1/1 -> pipeline20/1(d)
  pipeline20/1(q) -> local_time_lsw/1(out_reg)
  slice2/1 -> pipeline19/1(d)
  pipeline19/1(q) -> local_time_msw/1(out_reg)
  end_time_lsw/1(in_reg) -> pipeline28/1(d)
  end_time_msw/1(in_reg) -> pipeline27/1(d)
  start_time_lsw/1(in_reg) -> pipeline26/1(d)
  start_time_msw/1(in_reg) -> pipeline25/1(d)
  control_output/4(in_sample_end) -> pipeline24/1(d)
  control_output/3(in_sample_start) -> pipeline23/1(d)
  control_output/2(in_reset_en_time) -> pipeline22/1(d)
  control_output/1(in_load_en_time) -> pipeline21/1(d)
  bus_create/1(bus_out) -> pipeline29/1(d)
  receptor_id/2(in_pol0_id) -> pipeline30/1(d)
  receptor_id/3(in_pol1_id) -> pipeline31/1(d)
  flag_setup/1(in_adc_count) -> pipeline32/1(d)
  flag_setup/2(in_adc_flag) -> pipeline33/1(d)
  flag_setup/3(in_ndiode_flag) -> pipeline34/1(d)
  flag_setup/4(in_load_flags) -> pipeline35/1(d)
  flag_setup/5(in_reset_flags) -> pipeline36/1(d)
  pipeline36/1(q) -> edge_detect8/1(in)
  pipeline35/1(q) -> edge_detect9/1(in)
  pipeline34/1(q) -> [ndiode_flag]
  pipeline33/1(q) -> [adc_flag]
  pipeline32/1(q) -> [adc_count]
  start_flag_msw/1(in_reg) -> pipeline37/1(d)
  pipeline37/1(q) -> Concat4/1
  start_flag_lsw/1(in_reg) -> pipeline38/1(d)
  pipeline38/1(q) -> Concat4/2
  end_flag_msw/1(in_reg) -> pipeline39/1(d)
  pipeline39/1(q) -> Concat5/1
  end_flag_lsw/1(in_reg) -> pipeline40/1(d)
  pipeline40/1(q) -> Concat5/2
  pipeline53/1(q) -> bus_mult1/1(a), [cwg1_tp0]
  pipeline52/1(q) -> bus_mult1/2(b)
  pipeline51/1(q) -> bus_mult/2(b)
  pipeline54/1(q) -> Slice22/1, [spead_data0]
  pipeline55/1(q) -> Gateway Out22/1, [spead_valid0]
  pipeline56/1(q) -> [spead_eof0]
  pipeline57/1(q) -> [spead_data1]
  pipeline58/1(q) -> [spead_valid1]
  pipeline59/1(q) -> [spead_eof1]
  pipeline60/1(q) -> [spead_data2]
  pipeline61/1(q) -> [spead_valid2]
  pipeline62/1(q) -> [spead_eof2]
  pipeline63/1(q) -> [spead_data3]
  pipeline64/1(q) -> [spead_valid3]
  pipeline65/1(q) -> [spead_eof3]
  [gbe_rst] -> pipeline66/1(d)
  pipeline66/1(q) -> gbe0/1(rst)
  [clr_status] -> pipeline67/1(d)
  pipeline67/1(q) -> gbe0/9(debug_rst)
  pipeline68/1(q) -> gbe1/1(rst)
  pipeline69/1(q) -> gbe1/9(debug_rst)
  pipeline70/1(q) -> gbe2/1(rst)
  pipeline71/1(q) -> gbe2/9(debug_rst)
  [gbe_rst] -> pipeline72/1(d)
  pipeline72/1(q) -> gbe3/1(rst)
  [clr_status] -> pipeline73/1(d)
  pipeline73/1(q) -> gbe3/9(debug_rst)
  pipeline86/1(q) -> gbe0/3(tx_valid)
  pipeline84/1(q) -> gbe0/6(tx_end_of_frame)
  pipeline85/1(q) -> gbe1/3(tx_valid)
  pipeline81/1(q) -> gbe1/6(tx_end_of_frame)
  pipeline82/1(q) -> gbe2/3(tx_valid)
  pipeline87/1(q) -> gbe2/6(tx_end_of_frame)
  pipeline74/1(q) -> gbe3/2(tx_data)
  pipeline75/1(q) -> gbe3/3(tx_valid)
  pipeline76/1(q) -> gbe3/6(tx_end_of_frame)
  pipeline78/1(q) -> bus_addsub/1(a)
  pipeline79/1(q) -> bus_addsub/2(b)
  pipeline88/1(q) -> bus_addsub1/1(a)
  wng_corr/1(bus_out) -> pipeline88/1(d), pipeline79/1(d)
  pipeline89/1(q) -> bus_addsub1/2(b)
  pipeline91/1(q) -> bus_addsub2/2(b)
  pipeline92/1(q) -> bus_addsub3/1(a)
  pipeline93/1(q) -> bus_addsub3/2(b)
  pipeline94/1(q) -> [cwg_80_0]
  pipeline95/1(q) -> [cwg_80_1]
  pipeline96/1(q) -> pack_80_64_00/1(data80)
  pipeline97/1(q) -> pack_80_64_00/2(valid80)
  pipeline98/1(q) -> pack_80_64_00/3(word_start)
  pipeline99/1(q) -> pack_80_64_00/4(pkt_start)
  pipeline100/1(q) -> pack_80_64_1/1(data80)
  pipeline101/1(q) -> pack_80_64_1/2(valid80)
  pipeline102/1(q) -> pack_80_64_1/3(word_start)
  pipeline103/1(q) -> pack_80_64_1/4(pkt_start)
  pipeline105/1(q) -> pack_80_64_2/2(valid80)
  pipeline104/1(q) -> pack_80_64_2/1(data80)
  pipeline106/1(q) -> pack_80_64_2/3(word_start)
  pipeline107/1(q) -> pack_80_64_2/4(pkt_start)
  pipeline108/1(q) -> pack_80_64_3/1(data80)
  pipeline109/1(q) -> pack_80_64_3/2(valid80)
  pipeline110/1(q) -> pack_80_64_3/3(word_start)
  pipeline111/1(q) -> pack_80_64_3/4(pkt_start)
  pipeline112/1(q) -> Gateway Out26/1, spead_pack0/1(data64_ready)
  pipeline113/1(q) -> Gateway Out25/1, spead_pack0/2(data64_valid)
  pipeline114/1(q) -> spead_pack0/3(data64), Slice23/1
  pipeline115/1(q) -> spead_pack1/1(data64_ready)
  pipeline116/1(q) -> spead_pack1/2(data64_valid)
  pipeline118/1(q) -> spead_pack2/1(data64_ready)
  pipeline119/1(q) -> spead_pack2/2(data64_valid)
  pipeline121/1(q) -> spead_pack3/1(data64_ready)
  pipeline122/1(q) -> spead_pack3/2(data64_valid)
  pipeline125/1(q) -> [gbe_port2]
  pipeline124/1(q) -> [gbe_port3]
  pipeline15/1(q) -> pipeline14/1(d), pipeline9/1(d)
  Delay2/1 -> bus_addsub4/2(b)
  Delay13/1 -> Logical8/1, Logical6/1
  Delay14/1 -> Logical7/2
  Delay15/1 -> Delay18/1
  Delay16/1 -> Delay19/1
  Delay17/1 -> Logical5/1
  Delay18/1 -> Delay20/1
  Delay19/1 -> Delay21/1
  Delay20/1 -> sample_masking/3(first_samples)
  Delay21/1 -> sample_masking/4(last_samples)
  Delay22/1 -> Logical3/2
  Delay23/1 -> Logical1/1
  Delay24/1 -> Delay25/1
  Delay25/1 -> Delay26/1
  Delay26/1 -> Delay27/1
  Delay27/1 -> sample_masking/1(timei)
  sample_masking/4(flag_valid) -> Delay28/1
  Delay28/1 -> [flag_en]
  Logical1/1 -> sample_masking/7(flag_en)  "flag_en"
  sample_masking/1(timeo) -> Delay29/1
  Delay29/1 -> [masked_time]
  [local_time] -> Delay30/1
  [en_armed] -> Delay31/1
  [local_time] -> Delay32/1, Delay34/1, Delay38/1, Delay40/1
  [start_time] -> Delay33/1
  [end_time] -> Delay35/1, Delay36/1
  Delay30/1 -> Delay24/1
  Delay31/1 -> Delay13/1
  Delay32/1 -> Relational3/1
  Delay33/1 -> Relational3/2
  Delay34/1 -> Relational4/1
  Delay35/1 -> Relational4/2
  Delay36/1 -> Relational5/1
  Delay37/1 -> Relational5/2
  Delay38/1 -> Relational6/1
  Delay39/1 -> Relational6/2
  Delay40/1 -> Relational7/1
  Delay41/1 -> Relational7/2
  Delay44/1 -> Logical4/1, Logical2/1
  Delay45/1 -> Relational/1
  Delay46/1 -> Relational/2
  Delay47/1 -> Relational1/1
  Delay48/1 -> Relational1/2
  Delay51/1 -> Relational2/1
  bus_convert/1(dout) -> [cwg0_tp2], pipeline94/1(d)
  Pulse Generator1/1 -> control/7(sim_7)
  pipeline49/1(q) -> cwg1/1(freq)
  bus_convert2/1(dout) -> [wng0_sum], Delay139/1
  bus_convert3/1(dout) -> [wng1_sum], Delay7/1
  bus_convert4/1(dout) -> Delay2/1
  bus_convert5/1(dout) -> Delay8/1
  bus_convert6/1(dout) -> pipeline50/1(d)
  bus_convert7/1(dout) -> pipeline53/1(d)
  Constant32/1 -> scale_wng1/1(sim_1)
  scale_wng0/1(in_scale) -> Gateway Out17/1, pipeline41/1(d)
  scale_out0/1(in_scale) -> Gateway Out5/1, pipeline51/1(d)
  pipeline127/1(q) -> [pol0_always_on]
  [pol0_always_on] -> gbe0_traffic_control/1(always_on)
  [pol0_requested_pkts] -> gbe0_traffic_control/2(requested_pkts)
  [pol0_offset_data] -> gbe0_traffic_control/3(offset_data)
  [mrst] -> gbe0_traffic_control/4(mrst)
  [pol0_traffic_trigger] -> gbe0_traffic_control/5(traffic_trigger)
  gbe0_traffic_control/1(gbe_txen_gate) -> [gbe_txen_gate0]
  Constant68/1 -> pol1_sample_offset/1(sim_1)
  pipeline129/1(q) -> [pol1_offset_data]
  Constant67/1 -> pol0_sample_offset/1(sim_1)
  pipeline128/1(q) -> [pol0_offset_data]
  Constant69/1 -> pol0_num_pkts/1(sim_1)
  pipeline126/1(q) -> [pol0_requested_pkts]
  Constant73/1 -> pol1_num_pkts/1(sim_1)
  pipeline134/1(q) -> [pol1_requested_pkts]
  pipeline136/1(q) -> [pol1_always_on]
  pipeline5/1(q) -> Terminator49/1
  Delay/1 -> pol_traffic_trigger/1(sim_1)
  Constant66/1 -> pol_tx_always_on/1(sim_1)
  Constant77/1 -> pol_tx_always_on/2(sim_2)
  pol0_num_pkts/1(in_pol0_num_pkts) -> pipeline126/1(d)
  pol1_num_pkts/1(in_pol1_num_pkts) -> pipeline134/1(d)
  pol_tx_always_on/1(in_pol0_tx_always_on) -> pipeline127/1(d)
  pol_tx_always_on/2(in_pol1_tx_always_on) -> pipeline136/1(d)
  pol0_sample_offset/1(in_pol0_sample_offset) -> pipeline128/1(d)
  pol1_sample_offset/1(in_pol1_sample_offset) -> pipeline129/1(d)
  Delay52/1 -> pol_traffic_trigger/2(sim_2)
  pol_traffic_trigger/1(in_pol0_tx_trigger) -> pipeline131/1(d)
  pipeline130/1(q) -> [pol1_traffic_trigger]
  pol_traffic_trigger/2(in_pol1_tx_trigger) -> pipeline130/1(d)
  gbe2/4(tx_afull) -> Terminator28/1
  edge_detect3/1(out) -> Terminator50/1  "mrst"
  Constant64/1 -> freq_cwg0/1(sim_1)
  scale_cwg0/1(in_scale) -> pipeline44/1(d)
  freq_cwg0/1(in_frequency) -> pipeline45/1(d)
  Constant71/1 -> freq_cwg1/1(sim_1)
  freq_cwg1/1(in_frequency) -> pipeline49/1(d)
  Constant79/1 -> freq_cwg_corr/1(sim_1)
  freq_cwg_corr/1(in_frequency) -> pipeline47/1(d)
  scale_cwg_corr/1(in_scale) -> pipeline46/1(d)
  AddSub/1 -> Slice/1
  AddSub1/1 -> Slice1/1
  [tvg_stime] -> AddSub1/1, AddSub/1
  Constant81/1 -> speadtime0_offset/1(sim_1)
  Slice/1 -> Register5/1
  Slice1/1 -> Register6/1
  speadtime0_offset/1(in_speadtime_offset0) -> AddSub/2
  Constant82/1 -> speadtime1_offset/1(sim_1)
  speadtime1_offset/1(in_speadtime_offset1) -> AddSub1/2
  [Bus_expand_cwg0] -> CWG_0_Out/1(In1)
  [Bus_expand_cwg1] -> CWG_1_Out/1(In1)
  pipeline131/1(q) -> [pol0_traffic_trigger]
  Constant37/1 -> scale_cwg0/1(sim_1)
  Constant72/1 -> scale_cwg0/2(sim_2)
  Constant41/1 -> scale_cwg1/1(sim_1)
  Constant75/1 -> scale_cwg1/2(sim_2)
  scale_cwg1/1(in_scale) -> pipeline48/1(d)
  Constant80/1 -> scale_cwg_corr/1(sim_1)
  Constant78/1 -> scale_cwg_corr/2(sim_2)
  Constant58/1 -> scale_out1/1(sim_1)
  Constant63/1 -> scale_out1/2(sim_2)
  scale_out1/2(in_dummy) -> Terminator51/1
  Constant57/1 -> scale_out0/1(sim_1)
  Constant61/1 -> scale_out0/2(sim_2)
  scale_out0/2(in_dummy) -> Terminator/1
  gbe1_traffic_control/1(gbe_txen_gate) -> [gbe_txen_gate1]
  gbe2_traffic_control/1(gbe_txen_gate) -> [gbe_txen_gate2]
  gbe3_traffic_control/1(gbe_txen_gate) -> [gbe_txen_gate3]
  [spead_valid1] -> Logical9/1
  edge_detect7/1(out) -> pipeline132/1(d)
  [spead_valid0] -> edge_detect7/1(in)
  pipeline132/1(q) -> Register4/2
  [spead_data0] -> Register4/1
  Gateway Out9/1 -> To Workspace9/1
  Register4/1 -> Slice5/1
  Slice5/1 -> Gateway Out9/1
  [spead_valid0] -> gbe0_traffic_control/6(spead_valid)
  [pol0_always_on] -> gbe1_traffic_control/1(always_on)
  [pol0_requested_pkts] -> gbe1_traffic_control/2(requested_pkts)
  [pol0_offset_data] -> gbe1_traffic_control/3(offset_data)
  [mrst] -> gbe1_traffic_control/4(mrst)
  [pol0_traffic_trigger] -> gbe1_traffic_control/5(traffic_trigger)
  [pol1_always_on] -> gbe2_traffic_control/1(always_on)
  [pol1_requested_pkts] -> gbe2_traffic_control/2(requested_pkts)
  [pol1_offset_data] -> gbe2_traffic_control/3(offset_data)
  [mrst] -> gbe2_traffic_control/4(mrst)
  [pol1_traffic_trigger] -> gbe2_traffic_control/5(traffic_trigger)
  [pol1_always_on] -> gbe3_traffic_control/1(always_on)
  [pol1_requested_pkts] -> gbe3_traffic_control/2(requested_pkts)
  [pol1_offset_data] -> gbe3_traffic_control/3(offset_data)
  [mrst] -> gbe3_traffic_control/4(mrst)
  [pol1_traffic_trigger] -> gbe3_traffic_control/5(traffic_trigger)
  [spead_valid1] -> gbe1_traffic_control/6(spead_valid)
  [spead_valid2] -> gbe2_traffic_control/6(spead_valid)
  [spead_valid3] -> gbe3_traffic_control/6(spead_valid)
  Constant59/1 -> Delay/1
  Constant40/1 -> Delay52/1
  master_reset_sim7/1 -> dram_addr_offset/1(sim_1)
  master_reset_sim8/1 -> arb_rst/1(sim_1)
  master_reset_sim9/1 -> arb_en/1(sim_1)
  pipeline133/1(q) -> [arb_en0]
  pipeline138/1(q) -> [dram_addr_offset0]
  master_reset_sim1/1 -> dram_read_length/1(sim_1)
  master_reset_sim2/1 -> dram_rd_trigger/1(sim_1)
  pipeline150/1(q) -> [dram_rd_trig0]
  master_reset_sim3/1 -> dram_tvg/1(sim_1)
  master_reset_sim4/1 -> dram_tvg_length/1(sim_1)
  pipeline148/1(q) -> [dram_tvg_length0]
  edge_detect13/1(out) -> [arb_rst0]
  pipeline135/1(q) -> edge_detect13/1(in)
  master_reset_sim5/1 -> dram_rd_repeat/1(sim_1)
  pipeline151/1(q) -> [dram_rd_repeat0]
  pipeline146/1(q) -> Slice13/1, Slice11/1
  Slice13/1 -> Logical17/1, [tvg_sel0]
  Slice11/1 -> Logical17/2
  Logical17/1 -> [dram_tvg0]
  pipeline149/1(q) -> [dram_read_length0]
  master_reset_sim6/1 -> dram_rd_repeat_rate/1(sim_1)
  pipeline137/1(q) -> [dram_rd_repeat_delay0]
  [cwg_80_1] -> pipeline193/1(d)
  [cwg_80_0] -> pipeline190/1(d)
  pipeline158/1(q) -> [source_sel_0]
  pipeline159/1(q) -> [source_sel_1]
  Constant87/1 -> src_sel_cntrl/1(sim_1)
  Constant88/1 -> src_sel_cntrl/2(sim_2)
  src_sel_cntrl/1(in_src_sel_0) -> pipeline158/1(d)
  src_sel_cntrl/2(in_src_sel_1) -> pipeline159/1(d)
  [source_sel_0] -> pipeline189/1(d)
  [source_sel_1] -> pipeline192/1(d)
  Gateway Out40/1 -> To Workspace40/1
  Inverter/1 -> Gateway Out40/1, fifo1/2(fifo_we_en)
  Mux5/1 -> pipeline195/1(d)
  Mux4/1 -> pipeline196/1(d)
  Gateway Out1/1 -> To Workspace1/1
  Logical18/1 -> Inverter/1, fifo0/2(fifo_we_en), [fifoselect], Gateway Out1/1
  Gateway Out4/1 -> To Workspace4/1
  master_reset_sim10/1 -> arb_rst/2(sim_2)
  master_reset_sim11/1 -> dram_rd_trigger/2(sim_2)
  master_reset_sim12/1 -> arb_en/2(sim_2)
  Gateway Out21/1 -> To Workspace21/1
  Slice22/1 -> Gateway Out21/1
  Gateway Out22/1 -> To Workspace22/1
  Gateway Out23/1 -> To Workspace23/1
  Gateway Out24/1 -> To Workspace24/1
  Slice23/1 -> Gateway Out24/1
  Gateway Out25/1 -> To Workspace25/1
  Gateway Out26/1 -> To Workspace26/1
  dram_rd_repeat_rate/1(in_dram_rd_repeat_rate) -> pipeline137/1(d)
  dram_rd_repeat/1(in_dram_rd_repeat) -> pipeline151/1(d)
  dram_tvg/1(in_arb_tvg) -> pipeline146/1(d)
  dram_tvg_length/1(in_tvg_length) -> pipeline148/1(d)
  dram_addr_offset/1(in_dram_addr_offset) -> pipeline138/1(d)
  dram_read_length/1(in_dram_read_length) -> pipeline149/1(d)
  dram_rd_trigger/1(in_arb_trig) -> pipeline150/1(d)
  dram_rd_trigger/2(in_dummy) -> Terminator55/1
  arb_en/1(in_arb_en) -> pipeline133/1(d)
  arb_en/2(in_dummy) -> Terminator53/1
  arb_rst/1(in_rst) -> pipeline135/1(d)
  arb_rst/2(in_dummy) -> Terminator54/1
  pipeline189/1(q) -> Mux5/1
  pipeline190/1(q) -> Mux5/2
  pipeline191/1(q) -> Mux5/3
  pipeline192/1(q) -> Mux4/1
  pipeline193/1(q) -> Mux4/2
  pipeline194/1(q) -> Mux4/3
  pipeline45/1(q) -> cwg0/1(freq)
  pipeline44/1(q) -> cwg0/2(scale)
  [mrst] -> pipeline180/1(d)
  Constant60/1 -> rpt_en_cwg0/1(sim_1)
  Constant62/1 -> rpt_length_cwg0/1(sim_1)
  rpt_en_cwg0/2(in_dummy) -> Terminator57/1
  Constant70/1 -> rpt_en_cwg0/2(sim_2)
  rpt_en_cwg0/1(in_en) -> pipeline181/1(d)
  cwg0/1(bus_out) -> pipeline90/1(d), [Bus_expand_cwg0]
  cwg0/2(dvalid) -> [cwg0_dvalid]
  rpt_length_cwg0/1(in_cwg0_repeat_length) -> pipeline182/1(d)
  pipeline180/1(q) -> cwg0/3(rst)
  pipeline181/1(q) -> cwg0/4(repeat_en)
  pipeline182/1(q) -> cwg0/5(repeat_length)
  pipeline48/1(q) -> cwg1/2(scale)
  Constant76/1 -> rpt_en_cwg1/1(sim_1)
  rpt_en_cwg1/2(in_dummy) -> Terminator59/1
  Constant84/1 -> rpt_en_cwg1/2(sim_2)
  rpt_en_cwg1/1(in_en) -> pipeline183/1(d)
  pipeline183/1(q) -> cwg1/4(repeat_en)
  pipeline184/1(q) -> cwg1/5(repeat_length)
  [mrst] -> pipeline185/1(d)
  pipeline185/1(q) -> cwg1/3(rst)
  Constant83/1 -> rpt_length_cwg1/1(sim_1)
  rpt_length_cwg1/1(in_cwg1_repeat_length) -> pipeline184/1(d)
  [adc_count] -> Concat6/1
  Constant90/1 -> Concat6/2
  Delay4/1 -> [status0]
  Delay55/1 -> [status3]
  Delay54/1 -> [status2]
  Delay53/1 -> [status1]
  Concat6/1 -> Delay55/1, Delay4/1, Delay53/1, Delay54/1
  [ndiode_flag] -> Convert28/1
  Logical/1 -> Convert27/1
  Logical19/1 -> Convert30/1
  [adc_flag] -> Convert29/1
  [flag_en] -> Logical/1, Logical19/2
  Convert28/1 -> Logical/2
  Convert29/1 -> Logical19/1
  Convert30/1 -> Concat6/3
  Convert27/1 -> Concat6/4
  cwg0/3(rpt_rst) -> Terminator61/1
  pipeline198/1(q) -> wng0/2(rst)
  Constant23/1 -> man_rst_wng0/1(sim_1)
  Gateway Out12/1 -> To Workspace12/1
  Logical20/1 -> pipeline198/1(d)
  man_rst_wng0/1(in_rst) -> [wng0_man_rst], Logical20/2
  Gateway Out13/1 -> To Workspace13/1
  [wng0_rst] -> Logical20/1
  slice3/1 -> Gateway Out12/1
  [local_time] -> pipeline203/1(d)
  [mrst] -> pipeline201/1(d)
  [wng0_man_rst] -> pipeline199/1(d)
  wng_rst/1(wng_rst) -> Gateway Out13/1, [wng0_rst]
  Constant89/1 -> rpt_length_wng0/1(sim_1)
  pipeline200/1(q) -> wng_rst/5(num_samples_for_rst)
  pipeline199/1(q) -> wng_rst/4(man_rst)
  pipeline201/1(q) -> wng_rst/3(mrst)
  pipeline202/1(q) -> wng_rst/2(future_time)
  pipeline203/1(q) -> wng_rst/1(local_time)
  Constant95/1 -> rpt_load_time_msw_wng0/1(sim_1)
  Constant93/1 -> rpt_load_time_lsw_wng0/1(sim_1)
  Concat3/1 -> Delay1/1
  pipeline204/1(q) -> Concat3/1
  pipeline205/1(q) -> Concat3/2
  rpt_load_time_lsw_wng0/1(in_reg) -> pipeline205/1(d)
  rpt_load_time_msw_wng0/1(in_reg) -> pipeline204/1(d)
  Delay1/1 -> pipeline202/1(d)
  rpt_length_wng0/1(in_samples) -> pipeline206/1(d)
  pipeline206/1(q) -> pipeline200/1(d)
  [local_time] -> pipeline154/1(d)
  Impulse/1(impulse0) -> [Impulse_gen0]
  pipeline152/1(q) -> Impulse/2(future_time)
  pipeline154/1(q) -> Impulse/1(local_time)
  Constant92/1 -> impulse_load_time_msw/1(sim_1)
  Constant91/1 -> impulse_load_time_lsw/1(sim_1)
  Concat7/1 -> Delay10/1
  pipeline155/1(q) -> Concat7/1
  pipeline160/1(q) -> Concat7/2
  impulse_load_time_lsw/1(in_reg) -> pipeline160/1(d)
  impulse_load_time_msw/1(in_reg) -> pipeline155/1(d)
  Delay10/1 -> pipeline152/1(d)
  pipeline163/1(q) -> Mux5/4
  [Impulse_gen0] -> pipeline163/1(d)
  pipeline164/1(q) -> Mux4/4
  [Impulse_gen0] -> pipeline164/1(d)
  gpio/1 -> Terminator62/1
  Gateway Out/1 -> To Workspace/1
  Impulse/2(impulse_gpio) -> [Impulse_gpio]
  pipeline145/1(q) -> Impulse/3(delay_correction)
  impulse_delay_correction/1(in_reg) -> pipeline145/1(d)
  Constant55/1 -> impulse_delay_correction/1(sim_1)
  pipeline144/1(q) -> Gateway Out/1, gpio/1
  [Impulse_gpio] -> pipeline144/1(d)
  cwg1/3(rpt_rst) -> Terminator60/1
  cwg1/2(dvalid) -> Terminator63/1
  pipeline47/1(q) -> cwg_corr/1(freq)
  pipeline46/1(q) -> cwg_corr/2(scale)
  pipeline147/1(q) -> cwg_corr/3(rst)
  pipeline161/1(q) -> cwg_corr/4(repeat_en)
  pipeline162/1(q) -> cwg_corr/5(repeat_length)
  Constant96/1 -> cwg_corr/6(en)
  [mrst] -> pipeline147/1(d)
  rpt_en_cwg_corr/1(in_en) -> pipeline161/1(d)
  cwg_corr/3(rpt_rst) -> Terminator64/1
  cwg_corr/2(dvalid) -> Terminator65/1
  rpt_en_cwg_corr/2(in_dummy) -> Terminator78/1
  Constant97/1 -> rpt_en_cwg_corr/1(sim_1)
  Constant98/1 -> rpt_en_cwg_corr/2(sim_2)
  cwg_corr_repeat_length/1(in_cwg1_repeat_length) -> pipeline162/1(d)
  Constant99/1 -> cwg_corr_repeat_length/1(sim_1)
  [Bus_expand_cwg_corr] -> CWG_1_Out1/1(In1)
  [cwg_80_0] -> CWG_1_Out2/1(In1)
  pipeline50/1(q) -> [cwg0_tp0], bus_mult/1(a)
  [cwg_80_1] -> CWG_1_Out4/1(In1)
  pipeline165/1(q) -> wng1/2(rst)
  Logical21/1 -> pipeline165/1(d)
  man_rst_wng1/1(in_rst) -> Logical21/2
  [wng0_rst] -> Logical21/1
  Constant100/1 -> man_rst_wng1/1(sim_1)
  pipeline166/1(q) -> wng_corr/2(rst)
  Logical24/1 -> pipeline166/1(d)
  man_rst_wng_corr/1(in_rst) -> Logical24/2
  [wng0_rst] -> Logical24/1
  Constant101/1 -> man_rst_wng_corr/1(sim_1)
  Gateway Out3/1 -> To Workspace3/1
  Gateway Out5/1 -> To Workspace5/1
  bus_convert1/1(dout) -> [cwg1_tp2], pipeline95/1(d)
  Gateway Out6/1 -> To Workspace6/1
  Gateway Out17/1 -> To Workspace17/1
  Constant102/1 -> scale_wng1/2(sim_2)
  Constant103/1 -> scale_wng0/2(sim_2)
  Constant104/1 -> pipeline191/1(d)
  Constant105/1 -> pipeline194/1(d)
  [cwg1_tp2] -> bus_expand6/1(bus_in)
  [cwg1_tp0] -> bus_expand4/1(bus_in)
  [cwg0_tp2] -> bus_expand10/1(bus_in)
  [cwg0_tp0] -> bus_expand12/1(bus_in)
  [wng1_sum] -> bus_expand2/1(bus_in)
  [wng1_tp0] -> bus_expand8/1(bus_in)
  [wng0_tp0] -> bus_expand3/1(bus_in)
  [wng0_sum] -> bus_expand13/1(bus_in)
  [tvg_ltime] -> Delay11/1
  Delay11/1 -> Delay12/1
  [data_80_0] -> Delay56/1
  Delay56/1 -> Delay57/1
  bus_expand14/7(out2) -> pipeline167/1(d)
  bus_expand14/8(lsb_out1) -> pipeline170/1(d)
  bus_expand14/6(out3) -> pipeline171/1(d)
  bus_expand14/5(out4) -> pipeline172/1(d)
  bus_expand14/4(out5) -> pipeline209/1(d)
  bus_expand14/3(out6) -> pipeline210/1(d)
  bus_expand14/2(out7) -> pipeline211/1(d)
  bus_expand14/1(msb_out8) -> pipeline212/1(d)
  pipeline212/1(q) -> ss_fifo_in/1(in_d0)
  pipeline211/1(q) -> ss_fifo_in/2(in_d1)
  pipeline210/1(q) -> ss_fifo_in/3(in_d2)
  pipeline209/1(q) -> ss_fifo_in/4(in_d3)
  pipeline172/1(q) -> ss_fifo_in/5(in_d4)
  pipeline171/1(q) -> ss_fifo_in/6(in_d5)
  pipeline167/1(q) -> ss_fifo_in/7(in_d6)
  pipeline170/1(q) -> ss_fifo_in/8(in_d7)
  Delay57/1 -> bus_expand14/1(bus_in)
  Delay12/1 -> pipeline215/1(d), Relational8/1
  pipeline215/1(q) -> ss_localtime/1(in_time)
  pipeline213/1(q) -> ss_fifo_in/9(in_gpio_trig)
  Delay58/1 -> Delay59/1
  Delay59/1 -> pipeline213/1(d)
  [Impulse_gpio] -> Delay60/1
  Delay60/1 -> Delay58/1
  pipeline214/1(q) -> Impulse/4(Impulse_offset)
  Constant109/1 -> impulse_offset/1(sim_1)
  impulse_offset/1(in_reg) -> pipeline214/1(d)
  Constant108/1 -> ss_trig_time_msw/1(sim_1)
  Constant107/1 -> ss_trig_time_lsw/1(sim_1)
  Concat8/1 -> Delay61/1
  pipeline216/1(q) -> Concat8/1
  pipeline217/1(q) -> Concat8/2
  ss_trig_time_lsw/1(in_reg) -> pipeline217/1(d)
  ss_trig_time_msw/1(in_reg) -> pipeline216/1(d)
  Delay61/1 -> Relational8/2
  Relational8/1 -> edge_detect/1
  pipeline218/1(q) -> ss_fifo_in/10(we)
  [fifoselect] -> pipeline219/1(d), pipeline218/1(d)
  pipeline219/1(q) -> ss_localtime/2(we)
  edge_detect/1 -> ss_fifo_in/11(trig), ss_localtime/3(trig)
  Constant111/1 -> start_load_time_msw/1(sim_1)
  Constant110/1 -> start_load_time_lsw/1(sim_1)
  pipeline220/1(q) -> Concat9/1
  pipeline221/1(q) -> Concat9/2
  start_load_time_msw/1(in_reg) -> pipeline220/1(d)
  start_load_time_lsw/1(in_reg) -> pipeline221/1(d)
  Concat9/1 -> Delay62/1
  Constant113/1 -> stop_load_time_msw/1(sim_1)
  Constant112/1 -> stop_load_time_lsw/1(sim_1)
  pipeline222/1(q) -> Concat10/1
  pipeline223/1(q) -> Concat10/2
  stop_load_time_msw/1(in_reg) -> pipeline222/1(d)
  stop_load_time_lsw/1(in_reg) -> pipeline223/1(d)
  Concat10/1 -> Delay63/1
  Delay62/1 -> pipeline225/1(d)
  Delay63/1 -> pipeline224/1(d)
  pipeline225/1(q) -> Start_stop_Cntrl/1(start_time)
  pipeline224/1(q) -> Start_stop_Cntrl/2(stop_time)
  [mrst] -> Start_stop_Cntrl/3(rst)
  Start_stop_Cntrl/1(Start_Stop_Sel) -> [Start_Stop_Sel]
  pipeline195/1(q) -> Mux3/2
  Mux3/1 -> [data_80_0], bus_expand/1(bus_in)
  [Start_Stop_Sel] -> Mux3/1
  Mux6/1 -> bus_expand9/1(bus_in), [data_80_1]
  pipeline196/1(q) -> Mux6/2
  Constant114/1 -> Mux6/3
  [Start_Stop_Sel] -> Mux6/1
  Constant115/1 -> Mux3/3
  cwg1/1(bus_out) -> pipeline230/1(d)
  Constant74/1 -> cwg1/6(en)
  Constant106/1 -> cwg0/6(en)
  pipeline230/1(q) -> [Bus_expand_cwg1], pipeline93/1(d)
  pipeline90/1(q) -> bus_addsub2/1(a)
  tick_offset_msw/1(in_reg) -> pipeline17/1(d)
  pipeline117/1(q) -> spead_pack1/3(data64)
  pipeline120/1(q) -> spead_pack2/3(data64)
  pipeline123/1(q) -> spead_pack3/3(data64)
